simulink model "Bixler"  (R2019b)
settings: Solver=ode45  StartTime=0.0  StopTime=60  RelTol=1e-6  AbsTol=1e-8
PostLoadFcn:
  | parameters_main
  | write_init_cond
StartFcn:
  | write_init_cond
  | disp('Simulating...');
StopFcn:
  | timetime = datestr(datetime('now','Format','hh:mm'));
  | disp(['End of Simulation.       ', timetime]);
  | clear timetime
undefined symbols (not defined in the file): Aero, APlane, Bxl, C, Ctr, deg, DiscIntNeverNeededParam, Earth, F, Guid, Init, Light, MIL, Path, rad, s, Trim, Utility, WGS84
libraries: aerolibconvert2 x39, simulink x14, dspsigops x6, simulink_extras x3, aerolibtransform2 x2, aerolibasang x2, aerolibfltsims x2, shared6dof x1, aerolibadyn x1, aerolibwind2 x1, aerolibanim x1, realtime_pacer_lib x1
(part 1 of 5)
settings Model: SimulationMode=accelerator  PauseTimes=22.8  NumberOfSteps=10  Creator=extra  LastModifiedBy=YK
settings SolverCC: AutoScaleAbsTol=off
settings DataIOCC: SaveFormat=Array  SaveOutput=off  SignalLogging=off  DSMLogging=off  SaveTime=off  ReturnWorkspaceOutputs=off
settings OptimizationCC: EfficientMapNaN2IntZero=off
settings DebuggingCC: ReadBeforeWriteMsg=DisableAll  WriteAfterWriteMsg=DisableAll  WriteAfterReadMsg=DisableAll  MultiTaskDSMMsg=none  ArithmeticOperatorsInVariantConditions=warning
settings HardwareCC: TargetBitPerPointer=64  TargetBitPerSizeT=64  TargetBitPerPtrDiffT=64  TargetLongLongMode=on  TargetIntDivRoundTo=Zero  TargetEndianess=LittleEndian  TargetWordSize=64  TargetHWDeviceType=MATLAB Host  ProdEqTarget=off
settings ModelReferenceCC: UpdateModelReferenceTargets=IfOutOfDate
settings SFSimCC: SimUseLocalCustomCode=off  CustomCodeUndefinedFunction=UseInterfaceOnly
settings RTWCC: RTWUseLocalCustomCode=off
settings CodeAppCC: MaxIdLength=128  StateflowObjectComments=on
settings GRTTargetCC: TargetLangStandard=C89/C90 (ANSI)  CombineOutputUpdateFcns=off  GRTInterface=on
settings SimscapeCC: SimscapeNormalizeSystem=off

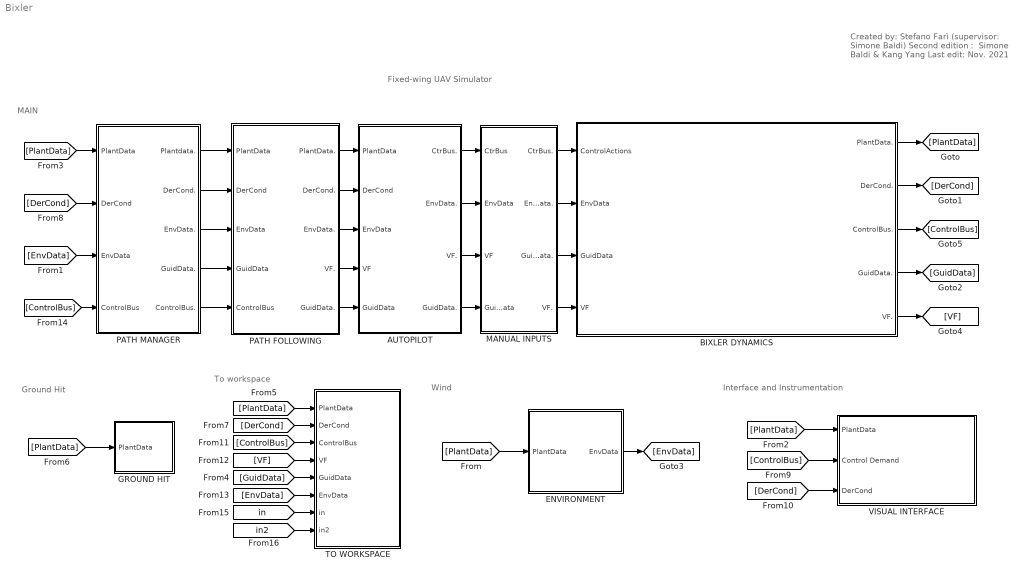
== system Bixler ==
  note: Fixed-wing UAV Simulator
  note: Ground Hit
  note: Interface and Instrumentation
  note: Wind
  note: MAIN
  note: To workspace
  note: Created by: Stefano Farì (supervisor: Simone Baldi)
      | Second edition： Simone Baldi & Kang Yang
      | Last edit: Nov. 2021
  AUTOPILOT : Subsystem
  BIXLER DYNAMICS : Subsystem
      mask Display: image('images/bixler.jpg')
  ENVIRONMENT : Subsystem
  GROUND HIT : Subsystem
  MANUAL INPUTS : Subsystem
  PATH FOLLOWING : Subsystem
  PATH MANAGER : Subsystem
  TO WORKSPACE : Subsystem
  VISUAL INTERFACE : Subsystem
      mask Display: image('images/control_tower.jpg')
  wires:
  BIXLER DYNAMICS/1(PlantData.) -> [PlantData]
  BIXLER DYNAMICS/2(DerCond.) -> [DerCond]
  [PlantData] -> ENVIRONMENT/1(PlantData)
  ENVIRONMENT/1(EnvData) -> [EnvData]
  [PlantData] -> VISUAL INTERFACE/1(PlantData)
  [ControlBus] -> VISUAL INTERFACE/2(Control Demand)
  PATH FOLLOWING/2("DerCond. ") -> AUTOPILOT/2(DerCond)
  PATH FOLLOWING/1("PlantData. ") -> AUTOPILOT/1(PlantData)
  [DerCond] -> VISUAL INTERFACE/3(DerCond)
  MANUAL INPUTS/1(CtrBus.) -> BIXLER DYNAMICS/1(ControlActions)
  [PlantData] -> TO WORKSPACE/1(PlantData)
  [PlantData] -> PATH MANAGER/1(PlantData)
  [DerCond] -> PATH MANAGER/2(DerCond)
  [PlantData] -> GROUND HIT/1(PlantData)
  MANUAL INPUTS/2(EnvData.) -> BIXLER DYNAMICS/2(EnvData)
  [ControlBus] -> TO WORKSPACE/3(ControlBus)
  [DerCond] -> TO WORKSPACE/2(DerCond)
  BIXLER DYNAMICS/3(ControlBus.) -> [ControlBus]
  [EnvData] -> PATH MANAGER/3(EnvData)
  PATH FOLLOWING/4(VF.) -> AUTOPILOT/4(VF)
  PATH FOLLOWING/3(EnvData.) -> AUTOPILOT/3(EnvData)
  PATH FOLLOWING/5(GuidData.) -> AUTOPILOT/5(GuidData)
  AUTOPILOT/4(GuidData.) -> MANUAL INPUTS/4(GuidData)
  BIXLER DYNAMICS/4(GuidData.) -> [GuidData]
  MANUAL INPUTS/3(GuidData.) -> BIXLER DYNAMICS/3(GuidData)
  [GuidData] -> TO WORKSPACE/5(GuidData)
  MANUAL INPUTS/4(VF.) -> BIXLER DYNAMICS/4(VF)
  BIXLER DYNAMICS/5(VF.) -> [VF]
  [VF] -> TO WORKSPACE/4(VF)
  PATH MANAGER/3(EnvData.) -> PATH FOLLOWING/3(EnvData)
  PATH MANAGER/2(DerCond.) -> PATH FOLLOWING/2(DerCond)
  PATH MANAGER/1(Plantdata.) -> PATH FOLLOWING/1(PlantData)
  PATH MANAGER/4(GuidData.) -> PATH FOLLOWING/4(GuidData)
  [EnvData] -> TO WORKSPACE/6(EnvData)
  AUTOPILOT/3(VF.) -> MANUAL INPUTS/3(VF)
  AUTOPILOT/2(EnvData.) -> MANUAL INPUTS/2(EnvData)
  AUTOPILOT/1(CtrBus.) -> MANUAL INPUTS/1(CtrBus)
  [ControlBus] -> PATH MANAGER/4(ControlBus)
  PATH MANAGER/5(ControlBus.) -> PATH FOLLOWING/5(ControlBus)
  [in] -> TO WORKSPACE/7(in)
  [in2] -> TO WORKSPACE/8(in2)

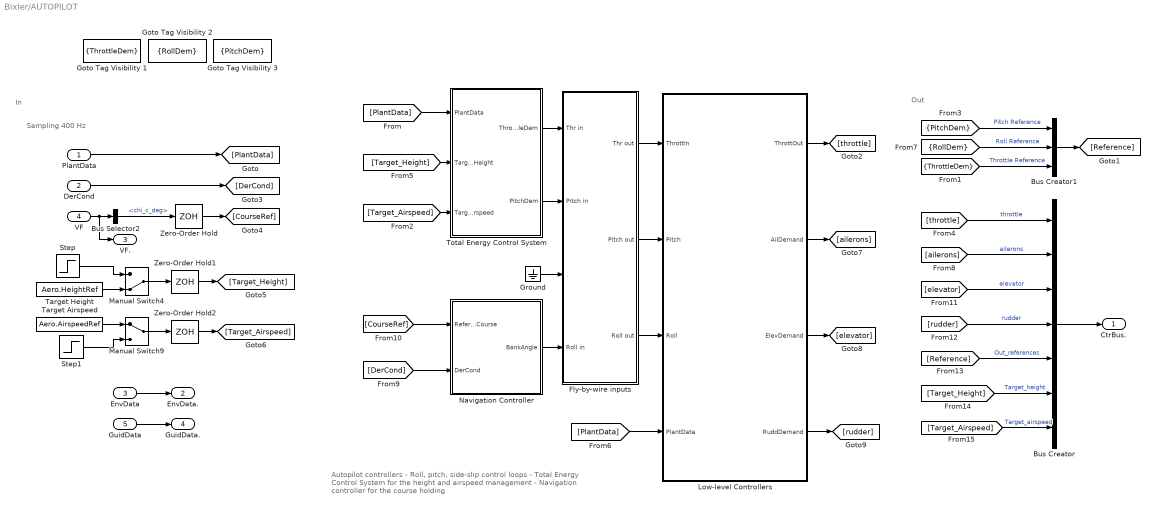
== system Bixler/AUTOPILOT ==
  note: In
  note: Out
  note: Autopilot controllers
      |
      | - Roll, pitch, side-slip control loops
      | - Total Energy Control System for the height and airspeed management
      | - Navigation controller for the course holding
  note: Sampling 400 Hz
  PlantData : Inport
  DerCond : Inport  Port=2
  EnvData : Inport  Port=3
  VF : Inport  Port=4
  GuidData : Inport  Port=5
  Bus Creator : BusCreator  Inputs=7
  Bus Creator1 : BusCreator  Inputs=3
  Bus Selector2 : BusSelector  OutputSignals=chi_c_deg
  Fly-by-wire inputs : Subsystem
  Goto Tag Visibility 1 : GotoTagVisibility  GotoTag=ThrottleDem
  Goto Tag Visibility 2 : GotoTagVisibility  GotoTag=RollDem
  Goto Tag Visibility 3 : GotoTagVisibility  GotoTag=PitchDem
  Ground : Ground
  Low-level Controllers : Subsystem
  Manual Switch4 : ManualSwitch  CurrentSetting=0
  Manual Switch9 : ManualSwitch
  Navigation Controller : Subsystem
  Step : Step  Time=10  Before=50  After=80  SampleTime=0
  Step1 : Step  Time=10  Before=15  After=20  SampleTime=0
  Target Airspeed : Constant  Value=Aero.AirspeedRef
  Target Height : Constant  Value=Aero.HeightRef
  Total Energy Control System : Subsystem
  Zero-Order Hold : ZeroOrderHold  SampleTime=1/400
  Zero-Order Hold1 : ZeroOrderHold  SampleTime=1/400
  Zero-Order Hold2 : ZeroOrderHold  SampleTime=1/400
  CtrBus. : Outport  VectorParamsAs1DForOutWhenUnconnected=off
  EnvData. : Outport  Port=2  VectorParamsAs1DForOutWhenUnconnected=off
  VF. : Outport  Port=3  VectorParamsAs1DForOutWhenUnconnected=off
  GuidData. : Outport  Port=4  VectorParamsAs1DForOutWhenUnconnected=off
  wires:
  Bus Creator1/1 -> [Reference]
  Low-level Controllers/4(RuddDemand) -> [rudder]
  Low-level Controllers/3(ElevDemand) -> [elevator]
  Low-level Controllers/2(AilDemand) -> [ailerons]
  Low-level Controllers/1(ThrottOut) -> [throttle]
  [RollDem] -> Bus Creator1/2  "Roll Reference"
  [CourseRef] -> Navigation Controller/1(ReferenceCourse)
  [PlantData] -> Low-level Controllers/4(PlantData)
  DerCond/1 -> [DerCond]
  [DerCond] -> Navigation Controller/2(DerCond)
  PlantData/1 -> [PlantData]
  Manual Switch4/1 -> Zero-Order Hold1/1
  Manual Switch9/1 -> Zero-Order Hold2/1
  Step/1 -> Manual Switch4/1
  Target Height/1 -> Manual Switch4/2
  Target Airspeed/1 -> Manual Switch9/1
  Step1/1 -> Manual Switch9/2
  [PitchDem] -> Bus Creator1/1  "Pitch Reference"
  Zero-Order Hold/1 -> [CourseRef]
  [PlantData] -> Total Energy Control System/1(PlantData)
  EnvData/1 -> EnvData./1
  GuidData/1 -> GuidData./1
  VF/1 -> VF./1, Bus Selector2/1
  Bus Selector2/1 -> Zero-Order Hold/1  "<chi_c_deg>"
  [ThrottleDem] -> Bus Creator1/3  "Throttle Reference"
  Zero-Order Hold1/1 -> [Target_Height]
  Zero-Order Hold2/1 -> [Target_Airspeed]
  Total Energy Control System/1(ThrottleDem) -> Fly-by-wire inputs/1(Thr in)
  Total Energy Control System/2(PitchDem) -> Fly-by-wire inputs/2(Pitch in)
  Navigation Controller/1(BankAngle) -> Fly-by-wire inputs/4(Roll in)
  Fly-by-wire inputs/1(Thr out) -> Low-level Controllers/1(ThrottIn)
  Fly-by-wire inputs/2(Pitch out) -> Low-level Controllers/2(Pitch)
  Fly-by-wire inputs/3(Roll out) -> Low-level Controllers/3(Roll)
  Ground/1 -> Fly-by-wire inputs/3(.)
  [Target_Height] -> Total Energy Control System/2(Target_Height)
  [Target_Airspeed] -> Total Energy Control System/3(Target_Airspeed)
  [ailerons] -> Bus Creator/2  "ailerons"
  [throttle] -> Bus Creator/1  "throttle"
  [elevator] -> Bus Creator/3  "elevator"
  [rudder] -> Bus Creator/4  "rudder"
  [Reference] -> Bus Creator/5  "Out_references"
  [Target_Height] -> Bus Creator/6  "Target_height"
  [Target_Airspeed] -> Bus Creator/7  "Target_airspeed"
  Bus Creator/1 -> CtrBus./1

== system Bixler/BIXLER DYNAMICS ==
  note: This sub-block contains the dynamics of the aircraft.
      |
      | - All the states and quantities of interest are contained in the Bus signal PlantData.
      | - The derived conditions such as Airspeed, Angle of Attack, and Side-slip angle, are contained in Bus signal DerCond .
      | - The Bus EnvData contains the wind quantities of interest.
      | - The dynamical model is continuous, but the Buses are sampled to feed the discrete-time control system.
      | - The parameters of this block are contained in parameters/parameters_aero.
  ControlActions : Inport
  EnvData : Inport  Port=2
  GuidData : Inport  Port=3
  VF : Inport  Port=4
  Actuator Dynamics : Subsystem
  Bus Selector : BusSelector  OutputSignals=throttle
  RUBBISH BIN : Subsystem
  Sampling : Subsystem
  "Sampling " : Subsystem
  Throttle Dynamics : Subsystem
  Vehicle Airframe : Subsystem
  PlantData. : Outport  VectorParamsAs1DForOutWhenUnconnected=off
  DerCond. : Outport  Port=2  VectorParamsAs1DForOutWhenUnconnected=off
  ControlBus. : Outport  Port=3  VectorParamsAs1DForOutWhenUnconnected=off
  GuidData. : Outport  Port=4  VectorParamsAs1DForOutWhenUnconnected=off
  VF. : Outport  Port=5  VectorParamsAs1DForOutWhenUnconnected=off
  wires:
  Vehicle Airframe/2(DerCond) -> "Sampling "/1(Cont.)  "DerCond"
  Bus Selector/1 -> Throttle Dynamics/1(In)  "<throttle>"
  EnvData/1 -> Vehicle Airframe/3(EnvData)
  ControlActions/1 -> Bus Selector/1, ControlBus./1, Actuator Dynamics/1(In)
  Vehicle Airframe/1(PlantData) -> Sampling/1(Cont.)  "PlantData"
  Sampling/1(Cont.+Disc.) -> PlantData./1
  "Sampling "/1(Cont.+Disc.) -> DerCond./1
  GuidData/1 -> GuidData./1
  VF/1 -> VF./1
  Actuator Dynamics/1(Out) -> Vehicle Airframe/2(ControlActions)
  Throttle Dynamics/1(Out) -> Vehicle Airframe/1(Throttle_cmd)  "throttle"

== system Bixler/ENVIRONMENT ==
  note: Wind slowly time varying
  note: Dynamic wind
  note: Constant wind
  PlantData : Inport
  Bus Creator : BusCreator  Inputs=4
  Bus Selector1 : BusSelector  OutputSignals=xyh,Velocity (inertial),From inertial to body matrix
  Bus Selector2 : BusSelector  OutputSignals=From inertial to body matrix
  Bus Selector3 : BusSelector  OutputSignals=PlantData
  Bus Selector4 : BusSelector  OutputSignals=From inertial to body matrix
  Constant1 : Constant  Value=Init.windConst
  Dot Product : DotProduct  InputSameDT=on  OutDataTypeStr=Inherit: Inherit via internal rule
  Dryden Wind Turbulence Model (Continuous (+q +r)) : aerolibwind2/Dryden Wind Turbulence Model  (Continuous (+q -r))  units=Metric (MKS)  spec=MIL-F-8785C  model=Continuous Dryden (+q +r)  W20=10  Wdeg=135  TurbProb=10^-2 - Light  L_high=533.4  Wingspan=Bxl.b  ts=0.1  Seed=[23341 23342 23343 23344]  T_on=on
  Height : Selector  InputPortWidth=3  IndexOptions=Index vector (dialog)  Indices=3  OutputSizes=1
  Init.DryOnOff : Gain  Gain=Init.DryOnOff
  "Init.DryOnOff " : Gain  Gain=Init.DryOnOff
  Init.WTimevar : Gain  Gain=Init.WTimevar
  Product : Product  Multiplication=Matrix(*)
  "Product " : Product  Multiplication=Matrix(*)
  Slowly time varying wind gen. : Subsystem
  Sum1 : Sum  Inputs=|++
  Sum3 : Sum  Inputs=|++
  Vt : Sqrt  SaturateOnIntegerOverflow=on
  EnvData : Outport  VectorParamsAs1DForOutWhenUnconnected=off
  wires:
  Bus Selector1/1 -> Height/1  "<xyh>"
  Bus Selector1/2 -> Dot Product/2, Dot Product/1  "<Velocity (inertial)>"
  Bus Selector1/3 -> Dryden Wind Turbulence Model (Continuous (+q +r))/3  "<From inertial to body matrix>"
  Bus Selector3/1 -> Bus Selector4/1, Bus Selector1/1, Bus Selector2/1  "<PlantData>"
  Height/1 -> Dryden Wind Turbulence Model (Continuous (+q +r))/1  "Altitude"
  Dot Product/1 -> Vt/1
  Vt/1 -> Dryden Wind Turbulence Model (Continuous (+q +r))/2  "Speed"
  Sum1/1 -> Bus Creator/3, Sum3/2  "Wind velocity (dyn) (body)"
  Constant1/1 -> Product/2
  Bus Creator/1 -> EnvData/1
  "Init.DryOnOff "/1 -> Bus Creator/4  "Wind ang rate (dyn) (body)"
  Sum3/1 -> Bus Creator/2  "Wind total (body)"
  Dryden Wind Turbulence Model (Continuous (+q +r))/1 -> Init.DryOnOff/1
  Bus Selector2/1 -> Product/1  "<From inertial to body matrix>"
  Dryden Wind Turbulence Model (Continuous (+q +r))/2 -> "Init.DryOnOff "/1
  PlantData/1 -> Bus Selector3/1
  Product/1 -> Bus Creator/1, Sum3/1  "Wind velocity (sta) (body)"
  Bus Selector4/1 -> "Product "/1  "<From inertial to body matrix>"
  Init.WTimevar/1 -> Sum1/2  "Wind slowly time varying"
  Init.DryOnOff/1 -> Sum1/1
  "Product "/1 -> Init.WTimevar/1
  Slowly time varying wind gen./1(Out1) -> "Product "/2

== system Bixler/GROUND HIT ==
  PlantData : Inport
  Bus Selector1 : BusSelector  OutputSignals=PlantData.xyh
  Constant : Constant  Value=0
  Relational Operator : RelationalOperator  Operator=<=  OutDataTypeStr=boolean  RndMeth=Simplest
  Selector : Selector  InputPortWidth=3  IndexOptions=Index vector (dialog)  Indices=3  OutputSizes=1
  Stop Simulation : Stop
  wires:
  Selector/1 -> Relational Operator/1
  Bus Selector1/1 -> Selector/1  "<xyh>"
  Constant/1 -> Relational Operator/2
  Relational Operator/1 -> Stop Simulation/1
  PlantData/1 -> Bus Selector1/1

== system Bixler/MANUAL INPUTS ==
  note: Manual control
      |
      | The switches below enable (up position) or disable (down position) the manual control in the Visual Interface sub-block.
      | (default: down)
  note: Open-loop inputs
      |
      | The switches below enables a custom input from the Workspace (timeseries data type) to the control surfaces.
  note: Trim condition
      |
      | The sub-block below allows to try the actuators configuration for a trimmed flight.
  CtrBus : Inport
  EnvData : Inport  Port=2
  VF : Inport  Port=3
  GuidData : Inport  Port=4
  Bus Creator : BusCreator  Inputs=7
  Bus Selector : BusSelector  OutputSignals=throttle,ailerons,elevator,rudder
  Bus Selector1 : BusSelector  OutputSignals=Out_references,Target_height,Target_airspeed
  "CtrBus " : InportShadow
  From Workspace1 : FromWorkspace  Commented=on  VariableName=LogData.RCIN.ElevDem_IN  SampleTime=0.001
  From Workspace2 : FromWorkspace  Commented=on  VariableName=LogData.RCIN.RuddDem_IN  SampleTime=0.001
  From Workspace3 : FromWorkspace  Commented=on  VariableName=LogData.RCIN.ThrottleDem_IN  SampleTime=0.001
  From Workspace4 : FromWorkspace  Commented=on  VariableName=LogData.RCIN.AilDem_IN  SampleTime=0.001
  Goto4 : Goto  Commented=on  GotoTag=throttle
  Manual Switch{,1..7} (8 alike) : ManualSwitch  CurrentSetting=0
  Manual_cmd{,4..6} (4 alike) : Constant  Value=0
  Trim conditions : Subsystem
  CtrBus. : Outport  VectorParamsAs1DForOutWhenUnconnected=off
  EnvData. : Outport  Port=2  VectorParamsAs1DForOutWhenUnconnected=off
  GuidData. : Outport  Port=3  VectorParamsAs1DForOutWhenUnconnected=off
  VF. : Outport  Port=4  VectorParamsAs1DForOutWhenUnconnected=off
  wires:
  Manual Switch4/1 -> Goto4/1, Bus Creator/1  "throttle"
  Manual Switch7/1 -> Bus Creator/3  "elevator"
  Manual_cmd/1 -> Manual Switch/1
  Manual_cmd4/1 -> Manual Switch1/1
  Manual Switch5/1 -> Bus Creator/2  "ailerons"
  Manual Switch6/1 -> Bus Creator/4  "rudder"
  Manual_cmd6/1 -> Manual Switch3/1
  Manual_cmd5/1 -> Manual Switch2/1
  Bus Creator/1 -> CtrBus./1
  Manual Switch1/1 -> Manual Switch5/2  "ailerons"
  Manual Switch2/1 -> Manual Switch7/2  "elevator"
  Manual Switch3/1 -> Manual Switch6/2  "rudder"
  From Workspace3/1 -> Manual Switch4/1
  Manual Switch/1 -> Manual Switch4/2
  Bus Selector/1 -> Trim conditions/1(throttle)  "<throttle>"
  Trim conditions/1(throttout) -> Manual Switch/2
  Bus Selector/2 -> Trim conditions/2(ail)  "<ailerons>"
  Bus Selector/3 -> Trim conditions/3(elev)  "<elevator>"
  Bus Selector/4 -> Trim conditions/4(rudd)  "<rudder>"
  Trim conditions/4(ruddout) -> Manual Switch3/2
  Trim conditions/2(ailout) -> Manual Switch1/2
  Trim conditions/3(elevout) -> Manual Switch2/2
  EnvData/1 -> EnvData./1
  From Workspace4/1 -> Manual Switch5/1
  From Workspace1/1 -> Manual Switch7/1
  From Workspace2/1 -> Manual Switch6/1
  GuidData/1 -> GuidData./1
  VF/1 -> VF./1
  CtrBus/1 -> Bus Selector/1
  "CtrBus "/1 -> Bus Selector1/1
  Bus Selector1/1 -> Bus Creator/5  "<Out_references>"
  Bus Selector1/2 -> Bus Creator/6  "<Target_height>"
  Bus Selector1/3 -> Bus Creator/7  "<Target_airspeed>"

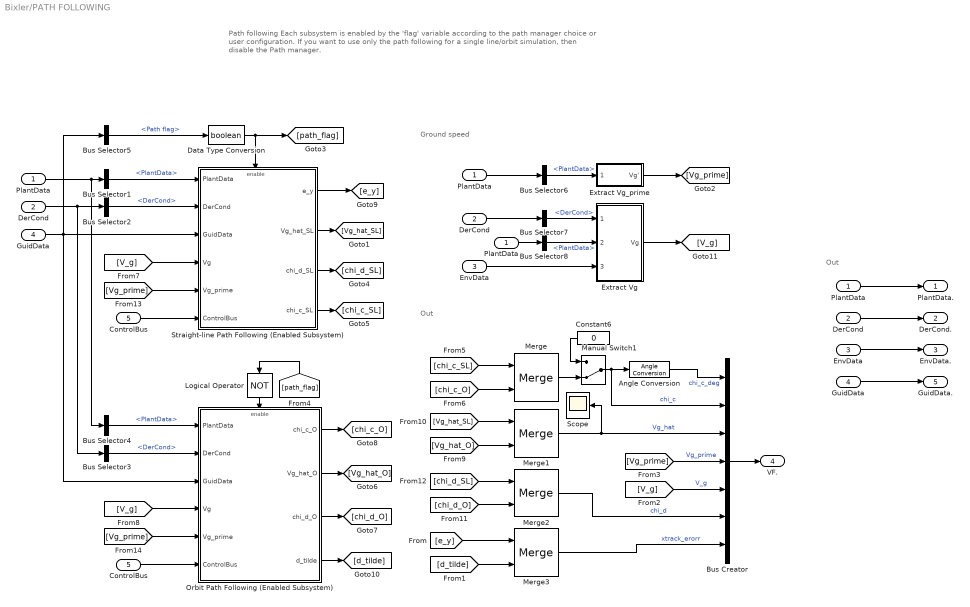
== system Bixler/PATH FOLLOWING ==
  note: Out
  note: Ground speed
  note: Out
  note: Path following
      |
      | Each subsystem is enabled by the 'flag' variable according to the path manager choice or user configuration.
      | If you want to use only the path following for a single line/orbit simulation, then disable the Path manager.
  PlantData : Inport
  DerCond : Inport  Port=2
  EnvData : Inport  Port=3
  GuidData : Inport  Port=4
  ControlBus : Inport  Port=5
  Angle Conversion : aerolibconvert2/Angle Conversion  IU=rad  OU=deg
  Bus Creator : BusCreator  Inputs=7
  Bus Selector{1,4,6,8} (4 alike) : BusSelector  OutputSignals=PlantData
  Bus Selector2 : BusSelector  OutputSignals=DerCond
  Bus Selector3 : BusSelector  OutputSignals=DerCond
  Bus Selector5 : BusSelector  OutputSignals=Path flag
  Bus Selector7 : BusSelector  OutputSignals=DerCond
  Constant6 : Constant  Value=0
  "ControlBus " : InportShadow  Port=5
  Data Type Conversion : DataTypeConversion  OutDataTypeStr=boolean
  "DerCond " : InportShadow  Port=2
  "DerCond  " : InportShadow  Port=2
  "EnvData " : InportShadow  Port=3
  Extract Vg : Subsystem
  Extract Vg_prime : Subsystem
  "GuidData " : InportShadow  Port=4
  Logical Operator : Logic  Operator=NOT  AllPortsSameDT=off  OutDataTypeStr=boolean
  Manual Switch1 : ManualSwitch  CurrentSetting=0
  Merge{,1..3} (4 alike) : Merge
  Orbit Path Following (Enabled Subsystem) : Subsystem  TreatAsAtomicUnit=on
  "PlantData " : InportShadow
  "PlantData  " : InportShadow
  "PlantData   " : InportShadow
  Scope : Scope
  Straight-line Path Following (Enabled Subsystem) : Subsystem  TreatAsAtomicUnit=on
  "PlantData. " : Outport  VectorParamsAs1DForOutWhenUnconnected=off
  "DerCond. " : Outport  Port=2  VectorParamsAs1DForOutWhenUnconnected=off
  EnvData. : Outport  Port=3  VectorParamsAs1DForOutWhenUnconnected=off
  VF. : Outport  Port=4  VectorParamsAs1DForOutWhenUnconnected=off
  GuidData. : Outport  Port=5  VectorParamsAs1DForOutWhenUnconnected=off
  wires:
  Merge/1 -> Manual Switch1/2
  Constant6/1 -> Manual Switch1/1
  EnvData/1 -> EnvData./1
  PlantData/1 -> Bus Selector4/1, Bus Selector1/1
  Bus Selector1/1 -> Straight-line Path Following (Enabled Subsystem)/1(PlantData)  "<PlantData>"
  DerCond/1 -> Bus Selector2/1, Bus Selector3/1
  Bus Creator/1 -> VF./1
  Manual Switch1/1 -> Bus Creator/2, Angle Conversion/1  "chi_c"
  Logical Operator/1 -> Orbit Path Following (Enabled Subsystem)/Enable
  Bus Selector4/1 -> Orbit Path Following (Enabled Subsystem)/1(PlantData)  "<PlantData>"
  Bus Selector3/1 -> Orbit Path Following (Enabled Subsystem)/2(DerCond)  "<DerCond>"
  Data Type Conversion/1 -> [path_flag], Straight-line Path Following (Enabled Subsystem)/Enable
  [path_flag] -> Logical Operator/1
  Bus Selector2/1 -> Straight-line Path Following (Enabled Subsystem)/2(DerCond)  "<DerCond>"
  Merge1/1 -> Bus Creator/3, Scope/1  "Vg_hat"
  [Vg_prime] -> Bus Creator/4  "Vg_prime"
  Straight-line Path Following (Enabled Subsystem)/2(Vg_hat_SL) -> [Vg_hat_SL]
  Straight-line Path Following (Enabled Subsystem)/3(chi_d_SL) -> [chi_d_SL]
  Straight-line Path Following (Enabled Subsystem)/4(chi_c_SL) -> [chi_c_SL]
  Orbit Path Following (Enabled Subsystem)/2(Vg_hat_O) -> [Vg_hat_O]
  Orbit Path Following (Enabled Subsystem)/3(chi_d_O) -> [chi_d_O]
  Orbit Path Following (Enabled Subsystem)/1(chi_c_O) -> [chi_c_O]
  [chi_c_SL] -> Merge/1
  [chi_c_O] -> Merge/2
  [Vg_hat_O] -> Merge1/2
  [Vg_hat_SL] -> Merge1/1
  [chi_d_O] -> Merge2/2
  [chi_d_SL] -> Merge2/1
  Merge2/1 -> Bus Creator/6  "chi_d"
  Angle Conversion/1 -> Bus Creator/1  "chi_c_deg"
  Straight-line Path Following (Enabled Subsystem)/1(e_y) -> [e_y]
  [e_y] -> Merge3/1
  Orbit Path Following (Enabled Subsystem)/4(d_tilde) -> [d_tilde]
  [d_tilde] -> Merge3/2
  Merge3/1 -> Bus Creator/7  "xtrack_erorr"
  GuidData/1 -> Orbit Path Following (Enabled Subsystem)/3(GuidData), Straight-line Path Following (Enabled Subsystem)/3(GuidData), Bus Selector5/1
  Bus Selector5/1 -> Data Type Conversion/1  "<Path flag>"
  "DerCond "/1 -> "DerCond. "/1
  "GuidData "/1 -> GuidData./1
  "PlantData "/1 -> "PlantData. "/1
  Extract Vg_prime/1(Vg') -> [Vg_prime]
  Bus Selector6/1 -> Extract Vg_prime/1(PlantData)  "<PlantData>"
  [V_g] -> Bus Creator/5  "V_g"
  Extract Vg/1(Vg) -> [V_g]
  "PlantData  "/1 -> Bus Selector6/1
  "DerCond  "/1 -> Bus Selector7/1
  Bus Selector7/1 -> Extract Vg/1(DerCond)  "<DerCond>"
  [V_g] -> Straight-line Path Following (Enabled Subsystem)/4(Vg)
  [V_g] -> Orbit Path Following (Enabled Subsystem)/4(Vg)
  [Vg_prime] -> Straight-line Path Following (Enabled Subsystem)/5(Vg_prime)
  [Vg_prime] -> Orbit Path Following (Enabled Subsystem)/5(Vg_prime)
  "EnvData "/1 -> Extract Vg/3(Envdata)
  ControlBus/1 -> Straight-line Path Following (Enabled Subsystem)/6(ControlBus)
  "ControlBus "/1 -> Orbit Path Following (Enabled Subsystem)/6(ControlBus)
  "PlantData   "/1 -> Bus Selector8/1
  Bus Selector8/1 -> Extract Vg/2(PlantData)  "<PlantData>"

== system Bixler/PATH MANAGER ==
  note: Change this switch to enable/disable the path manager (down = disabled).
  note: Path following only
  note: Path manager
  PlantData : Inport
  DerCond : Inport  Port=2
  EnvData : Inport  Port=3
  ControlBus : Inport  Port=4
  Bus Creator1 : BusCreator  Inputs=6
  Bus Creator2 : BusCreator  Inputs=6
  Bus Selector : BusSelector  OutputSignals=PlantData.Position (inertial)
  Constant1 : Constant  Value=Guid.SL.Line_Origin
  Constant10 : Constant  Value=Path.waypoints
  Constant2 : Constant  Value=Guid.Loiter.R
  Constant3 : Constant  Value=Guid.Loiter.R
  Constant4 : Constant  Value=Guid.SL.Line_Slope
  Constant5 : Constant  Value=Guid.Loiter.R
  Constant6 : Constant  Value=Guid.Loiter.C
  Constant7 : Constant  Value=Guid.Loiter.j
  Constant8 : Constant  Value=Guid.Strategy
  Demux : Demux  Outputs=2
  Manual Switch : ManualSwitch  CurrentSetting=0
  Path Manager : MATLAB Function  Commented=on  TreatAsAtomicUnit=on
  Scope : Scope
  Scope1 : Scope
  Selector2 : Selector  InputPortWidth=3  IndexOptions=Index vector (dialog)  Indices=[1 2]  OutputSizes=1
  Stop Simulation : Stop
  Plantdata. : Outport  VectorParamsAs1DForOutWhenUnconnected=off
  DerCond. : Outport  Port=2  VectorParamsAs1DForOutWhenUnconnected=off
  EnvData. : Outport  Port=3  VectorParamsAs1DForOutWhenUnconnected=off
  GuidData. : Outport  Port=4  VectorParamsAs1DForOutWhenUnconnected=off
  ControlBus. : Outport  Port=5  VectorParamsAs1DForOutWhenUnconnected=off
  wires:
  Constant8/1 -> Bus Creator1/1  "Path flag"
  Constant1/1 -> Bus Creator1/2  "SL_Origin"
  Constant4/1 -> Bus Creator1/3  "SL_Slope"
  Constant6/1 -> Bus Creator1/4  "Orbit_C"
  Constant5/1 -> Bus Creator1/5  "Orbit_R"
  Constant7/1 -> Bus Creator1/6  "Orbit_j"
  PlantData/1 -> Bus Selector/1, Plantdata./1
  DerCond/1 -> DerCond./1
  EnvData/1 -> EnvData./1
  Constant10/1 -> Path Manager/1(w)
  Bus Selector/1 -> Selector2/1  "<Position (inertial)>"
  Demux/1 -> Path Manager/2(x)
  Path Manager/6(stop_sim) -> Stop Simulation/1
  Selector2/1 -> Demux/1
  Demux/2 -> Path Manager/3(y)
  Bus Creator1/1 -> Manual Switch/2
  Manual Switch/1 -> GuidData./1
  Path Manager/7(z) -> Scope1/1
  Constant2/1 -> Path Manager/4(R)
  Bus Creator2/1 -> Manual Switch/1
  Path Manager/1(flag) -> Scope/1, Bus Creator2/1  "Path flag"
  Path Manager/2(origin) -> Bus Creator2/2  "SL_Origin"
  Path Manager/3(slope) -> Bus Creator2/3  "SL_Slope"
  Path Manager/4(c) -> Bus Creator2/4  "Orbit_C"
  Constant3/1 -> Bus Creator2/5  "Orbit_R"
  Path Manager/5(lambda) -> Bus Creator2/6  "Orbit_j"
  ControlBus/1 -> ControlBus./1

== system Bixler/TO WORKSPACE ==
  PlantData : Inport
  DerCond : Inport  Port=2
  ControlBus : Inport  Port=3
  VF : Inport  Port=4
  GuidData : Inport  Port=5
  EnvData : Inport  Port=6
  in : Inport  Port=7
  in2 : Inport  Port=8
  Bus Creator : BusCreator  Inputs=8
  Bus Selector4 : BusSelector  OutputSignals=DerCond
  Bus Selector5 : BusSelector  OutputSignals=PlantData
  Sample at 0.01s : ZeroOrderHold  SampleTime=0.01
  To Workspace2 : ToWorkspace  VariableName=SimOut  SaveFormat=Timeseries  SampleTime=-1
      settings: Save2DSignal=2-D array (concatenate along first dimension)
  wires:
  Bus Creator/1 -> Sample at 0.01s/1
  Bus Selector5/1 -> Bus Creator/1  "<PlantData>"
  PlantData/1 -> Bus Selector5/1
  ControlBus/1 -> Bus Creator/3  "ControlBus"
  DerCond/1 -> Bus Selector4/1
  Bus Selector4/1 -> Bus Creator/2  "<DerCond>"
  GuidData/1 -> Bus Creator/5  "GuidData"
  VF/1 -> Bus Creator/4  "VF"
  EnvData/1 -> Bus Creator/6  "EnvData"
  Sample at 0.01s/1 -> To Workspace2/1
  in/1 -> Bus Creator/7
  in2/1 -> Bus Creator/8

== system Bixler/VISUAL INTERFACE ==
  note: Position[m]:&nbsp;&nbsp;&nbsp;&nbsp;&nbsp;&nbsp;&nbsp;&nbsp;&nbsp;&nbsp;&nbsp;&nbsp;&nbsp;&nbsp;&nbsp;[0 0 -50]<br>Velocity[m/s]:&nbsp;&nbsp;&nbsp;&nbsp;&nbsp;&nbsp;&nbsp;&nbsp;&nbsp;&nbsp;&nbsp;&nbsp;&nbsp;[15 0 0]<br>Attitude[deg]:&nbsp;&nbsp;&nbsp;&nbsp;&nbsp;&nbsp;&nbsp;&nbsp;&nbsp;&nbsp;&nbsp;&nbsp;&nbsp;[0 0 0]<br>Angular rates[deg/s]:&nbsp;[0 0 0]<br><br>W. amplitude[m/s]:&nbsp;&nbsp;&nbsp;&nbsp;[-2 -3.4641 0]<br>
  note: Initial conditions
      | (Updates automatically)
  note: Extract data
  note: (remember to change the switch positions in the main block and to slow down the simulation with the Real-Time Parser)
  note: Actuators
  note: Positive, nose left-yawing
  note: Positive, right wing down
  note: Positive, nose down
  note: RUDDER
  note: AILERONS
  note: THROTTLE
  note: [m/s]
  note: [m]
  note: [m/s]
  note: ELEVATOR
  note: Slow down simulation to match
      | with real clock time
  PlantData : Inport
  Control Demand : Inport  Port=2
  DerCond : Inport  Port=3
  Ailerons : Display
  Airspeed Indicator : AirspeedIndicatorBlock  LabelPosition=Hide  ScaleMin=0  ScaleMax=40
  Altimeter : AltimeterBlock  LabelPosition=Hide
  Artificial Horizon : ArtificialHorizonBlock  LabelPosition=Hide
  Bus Selector : BusSelector  OutputSignals=Position (inertial),Euler angles (rad)
  Bus Selector1 : BusSelector  OutputSignals=PlantData
  Bus Selector2 : BusSelector  OutputSignals=DerCond
  Climb Rate Indicator : ClimbIndicatorBlock  LabelPosition=Hide  ScaleMax=20000
  Data for instrumentation below : Subsystem
  Elevator : Display
  Half Gauge : SemiCircularGaugeBlock  ScaleMin=-30  ScaleMax=30
  Half Gauge1 : SemiCircularGaugeBlock  ScaleMin=-30  ScaleMax=30
  Half Gauge2 : SemiCircularGaugeBlock  ScaleMin=-30  ScaleMax=30
  Half Gauge3 : SemiCircularGaugeBlock
  Heading Indicator : HeadingIndicatorBlock  LabelPosition=Hide
  MATLAB Animation : aerolibanim/MATLAB Animation  Tag=Matlab Animation 6 DOF  Vehicles=1  Geometries='astredwedge.mat'  BoundingBoxCoordinates=[-50,50,-50,50,-50,50]  CameraOffset=[-150,-50,0]  CameraViewAngle=3  SampleTime=0.2  FigurePosition=[6.189552e+01,5.544776e+01,6.039403e+02,5.444776e+02]
      settings: SourceProductBaseCode=AE
  Real-Time Pacer : realtime_pacer_lib/Real-Time Pacer  simTimePerRealTime=inf
  Rudder : Display
  Slider : SliderBlock
  Slider1 : SliderBlock  ScaleMin=-2  ScaleMax=2  TickInterval=1
  Slider2 : SliderBlock  ScaleMin=-1  ScaleMax=1  TickInterval=0.2
  Slider3 : SliderBlock  ScaleMin=-1  ScaleMax=1  TickInterval=0.2
  Subsystem : Subsystem
  Throttle : Display
  To FlightGear : Subsystem  Commented=on
  wires:
  Bus Selector/1 -> To FlightGear/1(In1), MATLAB Animation/1  "<Position (inertial)>"
  Bus Selector1/1 -> Data for instrumentation below/1(PlantData), Bus Selector/1  "<PlantData>"
  Bus Selector/2 -> To FlightGear/2(In2), MATLAB Animation/2  "<Euler angles (rad)>"
  Control Demand/1 -> Subsystem/1(Control Demand)
  Subsystem/1(t) -> Throttle/1
  Subsystem/2(e) -> Elevator/1
  Subsystem/3(a) -> Ailerons/1
  Subsystem/4(r) -> Rudder/1
  DerCond/1 -> Bus Selector2/1
  PlantData/1 -> Bus Selector1/1
  Bus Selector2/1 -> Data for instrumentation below/2(DerCond)  "<DerCond>"

== system Bixler/AUTOPILOT/Fly-by-wire inputs ==
  note: Put here your custom inputs
  Thr in : Inport
  Pitch in : Inport  Port=2
  . : Inport  Port=3
  Roll in : Inport  Port=4
  Constant : Constant  Commented=on  Value=0
  Dummy port : Terminator
  From Workspace : FromWorkspace  Commented=on  VariableName=LogData.RCIN.Throttle_IN  SampleTime=0.001
  From Workspace1 : FromWorkspace  Commented=on  VariableName=LogData.RCIN.Pitch_IN  SampleTime=0.001
  From Workspace2 : FromWorkspace  Commented=on  VariableName=LogData.RCIN.Roll_IN  SampleTime=0.001
  Manual Switch1 : ManualSwitch  CurrentSetting=0
  Manual Switch2 : ManualSwitch
  Manual Switch3 : ManualSwitch
  Manual Switch4 : ManualSwitch
  Thr out : Outport  VectorParamsAs1DForOutWhenUnconnected=off
  Pitch out : Outport  Port=2  VectorParamsAs1DForOutWhenUnconnected=off
  Roll out : Outport  Port=3  VectorParamsAs1DForOutWhenUnconnected=off
  tag scope: PitchDem=scoped, RollDem=scoped, ThrottleDem=scoped
  wires:
  Manual Switch3/1 -> Pitch out/1
  Manual Switch1/1 -> Thr out/1
  Pitch in/1 -> [PitchDem], Manual Switch3/1
  From Workspace/1 -> Manual Switch1/1
  Manual Switch2/1 -> [RollDem], Roll out/1
  Roll in/1 -> Manual Switch2/1
  From Workspace1/1 -> Manual Switch3/2
  Thr in/1 -> [ThrottleDem], Manual Switch1/2
  Constant/1 -> Manual Switch4/2
  From Workspace2/1 -> Manual Switch4/1
  Manual Switch4/1 -> Manual Switch2/2
  ./1 -> Dummy port/1

== system Bixler/AUTOPILOT/Low-level Controllers ==
  ThrottIn : Inport  Unit=%
  Pitch : Inport  Port=2  Unit=deg
  Roll : Inport  Port=3  Unit=deg
  PlantData : Inport  Port=4
  Angle Conversion1 : aerolibconvert2/Angle Conversion  IU=rad  OU=deg
  Angle Conversion2 : aerolibconvert2/Angle Conversion  IU=rad  OU=deg
  Angular Velocity Conversion : aerolibconvert2/Angular Velocity Conversion  IU=rad/s  OU=deg/s
  Angular Velocity Conversion1 : aerolibconvert2/Angular Velocity Conversion  IU=rad/s  OU=deg/s
  Bus Selector : BusSelector  OutputSignals=PlantData.Euler angles (rad)
  Bus Selector1 : BusSelector  OutputSignals=PlantData.Angular rates (body) (rad/s)
  Bus Selector2 : BusSelector  OutputSignals=PlantData.Euler angles (rad)
  Bus Selector3 : BusSelector  OutputSignals=PlantData.Angular rates (body) (rad/s)
  Bus Selector5 : BusSelector  OutputSignals=PlantData.Angular rates (body) (rad/s)
  Bus Selector6 : BusSelector  OutputSignals=PlantData.Euler angles (rad)
  Bus Selector7 : BusSelector  OutputSignals=PlantData.Accelerations (body/body)
  Get scaling factor : Subsystem
  Pitch controller : Subsystem
  Roll controller : Subsystem
  Side-slip angle controller : Subsystem
  ThrottOut : Outport  Unit=%  VectorParamsAs1DForOutWhenUnconnected=off
  AilDemand : Outport  Port=2  Unit=deg  VectorParamsAs1DForOutWhenUnconnected=off
  ElevDemand : Outport  Port=3  Unit=deg  VectorParamsAs1DForOutWhenUnconnected=off
  RuddDemand : Outport  Port=4  Unit=deg  VectorParamsAs1DForOutWhenUnconnected=off
  wires:
  Bus Selector/1 -> Angle Conversion1/1  "<Euler angles (rad)>"
  Roll controller/1(AilDemand) -> [AilDem], AilDemand/1
  Bus Selector1/1 -> Angular Velocity Conversion1/1  "<Angular rates (body) (rad/s)>"
  Bus Selector2/1 -> Angle Conversion2/1  "<Euler angles (rad)>"
  Bus Selector3/1 -> Angular Velocity Conversion/1  "<Angular rates (body) (rad/s)>"
  Pitch controller/1(ElevDemand) -> ElevDemand/1
  Get scaling factor/1(Scaler) -> Roll controller/4(Scaler), Side-slip angle controller/4(Scaler), Pitch controller/4(Scaler)
  Bus Selector7/1 -> Side-slip angle controller/3(accel_y)  "<Accelerations (body/body)>"
  Bus Selector6/1 -> Side-slip angle controller/2("Euler angles ")  "<Euler angles (rad)>"
  Bus Selector5/1 -> Side-slip angle controller/1(Yaw_rate)  "<Angular rates (body) (rad/s)>"
  [PlantData] -> Bus Selector1/1, Bus Selector2/1, Bus Selector3/1, Bus Selector5/1, Bus Selector6/1, Bus Selector7/1, Bus Selector/1
  Pitch/1 -> [PitchRef]
  PlantData/1 -> [PlantData]
  ThrottIn/1 -> ThrottOut/1
  Angle Conversion2/1 -> Pitch controller/2(EulerAngles)
  Angular Velocity Conversion/1 -> Pitch controller/3(AngularRates)
  Angle Conversion1/1 -> Roll controller/2(Euler angles)
  Angular Velocity Conversion1/1 -> Roll controller/3(AngularRates)
  Roll/1 -> [RollRef]
  [PitchRef] -> Pitch controller/1(PitchReference)
  [RollRef] -> Roll controller/1(RollReference)
  [AilDem] -> Side-slip angle controller/5(AilDemand)
  Side-slip angle controller/1(RudderDemand) -> RuddDemand/1

== system Bixler/AUTOPILOT/Navigation Controller ==
  ReferenceCourse : Inport  Unit=deg
  DerCond : Inport  Port=2
  Angle Conversion : aerolibconvert2/Angle Conversion  IU=rad  OU=deg
  Bus Selector : BusSelector  OutputSignals=DerCond.Course
  Constant : Constant  Value=45
  Discrete PID Controller : simulink/Continuous/PID Controller  Controller=PD  Form=Parallel  TimeDomain=Discrete-time  SampleTime=Ctr.TS  IntegratorMethod=Forward Euler  FilterMethod=Forward Euler  ControllerParametersSource=internal  P=Ctr.Hdg2Roll.NAV_ROLL_P  I=0.01  D=Ctr.Hdg2Roll.NAV_ROLL_D  UseFilter=on  N=2*pi*20  TunerSelectOption=Transfer Function Based (PID Tuner App)  InitialConditionSource=internal  InitialConditionForIntegrator=0  InitialConditionForFilter=0  DifferentiatorICPrevScaledInput=0  ExternalReset=none  TrackingMode=off  Kt=1  LimitOutput=on  UpperSaturationLimit=45  LowerSaturationLimit=-45  LinearizeAsGain=off  AntiWindupMode=clamping  Kb=1  POutMin=[]  POutMax=[]  IOutMin=[]  IOutMax=[]  DOutMin=[]  DOutMax=[]  NOutMin=[]  NOutMax=[]  SumOutMin=[]  SumOutMax=[]  SaturationOutMin=[]  SaturationOutMax=[]  PParamMin=[]  PParamMax=[]  IParamMin=[]  IParamMax=[]  DParamMin=[]  DParamMax=[]  NParamMin=[]  NParamMax=[]  KbParamMin=[]  KbParamMax=[]  KtParamMin=[]  KtParamMax=[]  KbOutMin=[]  KbOutMax=[]  KtOutMin=[]  KtOutMax=[]  IntegratorOutMin=[]  IntegratorOutMax=[]  FilterOutMin=[]  FilterOutMax=[]  SumI1OutMin=[]  SumI1OutMax=[]  SumI2OutMin=[]  SumI2OutMax=[]  SumI3OutMin=[]  SumI3OutMax=[]  SumI4OutMin=[]  SumI4OutMax=[]  SumDOutMin=[]  SumDOutMax=[]  DifferentiatorOutMin=[]  DifferentiatorOutMax=[]  FilterDiffOutCoefMin=[]  FilterDiffOutCoefMax=[]  ReciprocalOutMin=[]  ReciprocalOutMax=[]  SumDenOutMin=[]  SumDenOutMax=[]  SumNumOutMin=[]  SumNumOutMax=[]  DivideOutMin=[]  DivideOutMax=[]  IntegratorContinuousStateAttributes=''  IntegratorStateMustResolveToSignalObject=off  IntegratorRTWStateStorageClass=Auto  FilterContinuousStateAttributes=''  FilterStateMustResolveToSignalObject=off  FilterRTWStateStorageClass=Auto  ParallelPVariant=InternalParameters  IdealPVariant=Disabled  IVariant=Disabled  DVariant=InternalParameters  IntegratorVariant=Disabled  SatVariant=Enabled  AWVariant=Disabled  PCopyVariant=Disabled  TRVariant=Disabled  FdbkBlocksVariant=Forward  IdealPFdbkVariant=Disabled  SatFdbkVariant=Disabled  DerivativeFilterVariant=ForwardEulerFilter  NVariant=InternalParameters  NCopyVariant=Disabled  FilterICVariant=InternalICsFilter  IntegratorICVariant=Disabled  ExternalResetVariant=Disabled  TRSumVariant=Passthrough  SumFdbkVariant=Disabled  SumVariant=Sum_PD
  Manual Switch : ManualSwitch  CurrentSetting=0
  Manual Switch1 : ManualSwitch
  PID : Subsystem  Commented=on
  Scope : Scope
  Scope1 : Scope
  Scope2 : Scope  NumInputPorts=2
  Step : Step  Time=10  After=90  SampleTime=0
  Sum : Sum  Inputs=|+-
  Unwrap : Subsystem
  Unwrap1 : dspsigops/Unwrap  tol=pi  InputProcessing=Columns as channels (frame based)  running=off
  Zero-Order Hold : ZeroOrderHold  SampleTime=1/400
  BankAngle : Outport  Unit=deg  VectorParamsAs1DForOutWhenUnconnected=off
  wires:
  Bus Selector/1 -> Unwrap1/1  "<Course>"
  Discrete PID Controller/1 -> Manual Switch1/1, Scope/1
  DerCond/1 -> Bus Selector/1
  Unwrap1/1 -> Angle Conversion/1  "chi_measured"
  Sum/1 -> Scope1/1, Discrete PID Controller/1
  Angle Conversion/1 -> Sum/2, Scope2/2
  ReferenceCourse/1 -> Manual Switch/2
  Unwrap/1(Out) -> Scope2/1, Sum/1
  Manual Switch/1 -> Unwrap/1(In)
  Step/1 -> Zero-Order Hold/1
  Zero-Order Hold/1 -> Manual Switch/1
  Manual Switch1/1 -> BankAngle/1
  Constant/1 -> Manual Switch1/2

== system Bixler/AUTOPILOT/Total Energy Control System ==
  note: TECS (Total Energy Control System)
      |
      | It is meant to solve the cross-coupling between height and airspeed control. This is a simplified version of the TECS (see thesis for details). This implementation has the same theoretical behaviour of ArduPilot, but without a direct correspondence with its parameters.
  PlantData : Inport
  Target_Height : Inport  Port=2
  Target_Airspeed : Inport  Port=3
  Bus Selector1 : BusSelector  OutputSignals=PlantData.xyh
  Discrete PID Controller 1 : simulink/Continuous/PID Controller  Controller=PID  Form=Parallel  TimeDomain=Discrete-time  SampleTime=Ctr.TS  IntegratorMethod=Forward Euler  FilterMethod=Forward Euler  ControllerParametersSource=internal  P=1.73635676332661  I=0.34363794334664  D=0.534286386520939  UseFilter=on  N=1.11842208231346  TunerSelectOption=Transfer Function Based (PID Tuner App)  InitialConditionSource=internal  InitialConditionForIntegrator=0  InitialConditionForFilter=0  DifferentiatorICPrevScaledInput=0  ExternalReset=none  TrackingMode=off  Kt=1  LimitOutput=on  UpperSaturationLimit=100  LowerSaturationLimit=0  LinearizeAsGain=off  AntiWindupMode=clamping  Kb=1  POutMin=[]  POutMax=[]  IOutMin=[]  IOutMax=[]  DOutMin=[]  DOutMax=[]  NOutMin=[]  NOutMax=[]  SumOutMin=[]  SumOutMax=[]  SaturationOutMin=[]  SaturationOutMax=[]  PParamMin=[]  PParamMax=[]  IParamMin=[]  IParamMax=[]  DParamMin=[]  DParamMax=[]  NParamMin=[]  NParamMax=[]  KbParamMin=[]  KbParamMax=[]  KtParamMin=[]  KtParamMax=[]  KbOutMin=[]  KbOutMax=[]  KtOutMin=[]  KtOutMax=[]  IntegratorOutMin=[]  IntegratorOutMax=[]  FilterOutMin=[]  FilterOutMax=[]  SumI1OutMin=[]  SumI1OutMax=[]  SumI2OutMin=[]  SumI2OutMax=[]  SumI3OutMin=[]  SumI3OutMax=[]  SumI4OutMin=[]  SumI4OutMax=[]  SumDOutMin=[]  SumDOutMax=[]  DifferentiatorOutMin=[]  DifferentiatorOutMax=[]  FilterDiffOutCoefMin=[]  FilterDiffOutCoefMax=[]  ReciprocalOutMin=[]  ReciprocalOutMax=[]  SumDenOutMin=[]  SumDenOutMax=[]  SumNumOutMin=[]  SumNumOutMax=[]  DivideOutMin=[]  DivideOutMax=[]  IntegratorContinuousStateAttributes=''  IntegratorStateMustResolveToSignalObject=off  IntegratorRTWStateStorageClass=Auto  FilterContinuousStateAttributes=''  FilterStateMustResolveToSignalObject=off  FilterRTWStateStorageClass=Auto  ParallelPVariant=InternalParameters  IdealPVariant=Disabled  IVariant=InternalParameters  DVariant=InternalParameters  IntegratorVariant=Discrete  SatVariant=Enabled  AWVariant=DiscClampingParallel  PCopyVariant=Disabled  TRVariant=Disabled  FdbkBlocksVariant=Forward  IdealPFdbkVariant=Disabled  SatFdbkVariant=Disabled  DerivativeFilterVariant=ForwardEulerFilter  NVariant=InternalParameters  NCopyVariant=Disabled  FilterICVariant=InternalICsFilter  IntegratorICVariant=InternalICs  ExternalResetVariant=Disabled  TRSumVariant=Passthrough  SumFdbkVariant=Disabled  SumVariant=Sum_PID
  Discrete PID Controller 2 : simulink/Continuous/PID Controller  Controller=PID  Form=Parallel  TimeDomain=Discrete-time  SampleTime=Ctr.TS  IntegratorMethod=Forward Euler  FilterMethod=Forward Euler  ControllerParametersSource=internal  P=0.0957032759552278  I=0.0036993820124705  D=0.00128202697815644  UseFilter=on  N=46.36307138661  TunerSelectOption=Transfer Function Based (PID Tuner App)  InitialConditionSource=internal  InitialConditionForIntegrator=0  InitialConditionForFilter=0  DifferentiatorICPrevScaledInput=0  ExternalReset=none  TrackingMode=off  Kt=1  LimitOutput=on  UpperSaturationLimit=30  LowerSaturationLimit=-30  LinearizeAsGain=off  AntiWindupMode=clamping  Kb=1  POutMin=[]  POutMax=[]  IOutMin=[]  IOutMax=[]  DOutMin=[]  DOutMax=[]  NOutMin=[]  NOutMax=[]  SumOutMin=[]  SumOutMax=[]  SaturationOutMin=[]  SaturationOutMax=[]  PParamMin=[]  PParamMax=[]  IParamMin=[]  IParamMax=[]  DParamMin=[]  DParamMax=[]  NParamMin=[]  NParamMax=[]  KbParamMin=[]  KbParamMax=[]  KtParamMin=[]  KtParamMax=[]  KbOutMin=[]  KbOutMax=[]  KtOutMin=[]  KtOutMax=[]  IntegratorOutMin=[]  IntegratorOutMax=[]  FilterOutMin=[]  FilterOutMax=[]  SumI1OutMin=[]  SumI1OutMax=[]  SumI2OutMin=[]  SumI2OutMax=[]  SumI3OutMin=[]  SumI3OutMax=[]  SumI4OutMin=[]  SumI4OutMax=[]  SumDOutMin=[]  SumDOutMax=[]  DifferentiatorOutMin=[]  DifferentiatorOutMax=[]  FilterDiffOutCoefMin=[]  FilterDiffOutCoefMax=[]  ReciprocalOutMin=[]  ReciprocalOutMax=[]  SumDenOutMin=[]  SumDenOutMax=[]  SumNumOutMin=[]  SumNumOutMax=[]  DivideOutMin=[]  DivideOutMax=[]  IntegratorContinuousStateAttributes=''  IntegratorStateMustResolveToSignalObject=off  IntegratorRTWStateStorageClass=Auto  FilterContinuousStateAttributes=''  FilterStateMustResolveToSignalObject=off  FilterRTWStateStorageClass=Auto  ParallelPVariant=InternalParameters  IdealPVariant=Disabled  IVariant=InternalParameters  DVariant=InternalParameters  IntegratorVariant=Discrete  SatVariant=Enabled  AWVariant=DiscClampingParallel  PCopyVariant=Disabled  TRVariant=Disabled  FdbkBlocksVariant=Forward  IdealPFdbkVariant=Disabled  SatFdbkVariant=Disabled  DerivativeFilterVariant=ForwardEulerFilter  NVariant=InternalParameters  NCopyVariant=Disabled  FilterICVariant=InternalICsFilter  IntegratorICVariant=InternalICs  ExternalResetVariant=Disabled  TRSumVariant=Passthrough  SumFdbkVariant=Disabled  SumVariant=Sum_PID
  Fcn2 : Fcn  Expr=0.5 * u(1)^2
  Fcn4 : Fcn  Expr=0.5 * u(1)^2
  Gain1 : Gain  Gain=C.g
  Gain3 : Gain  Gain=C.g
  Selector1 : Selector  InputPortWidth=3  IndexOptions=Index vector (dialog)  Indices=3  OutputSizes=1
  Sum : Sum  Inputs=|++
  Sum11 : Sum  Inputs=+-
  Sum12 : Sum  Inputs=+-
  Sum13 : Sum  Inputs=|-+
  Sum8 : Sum  Inputs=|++
  Sum9 : Sum  Inputs=|-+
  ThrottleDem : Outport  VectorParamsAs1DForOutWhenUnconnected=off
  PitchDem : Outport  Port=2  VectorParamsAs1DForOutWhenUnconnected=off
  wires:
  Discrete PID Controller 2/1 -> PitchDem/1  "pitch"
  Discrete PID Controller 1/1 -> ThrottleDem/1  "throttle"
  [Va] -> Fcn2/1
  Fcn2/1 -> Sum/2, Sum11/2  "SKE"
  PlantData/1 -> Bus Selector1/1
  Bus Selector1/1 -> Selector1/1  "<xyh>"
  Selector1/1 -> Gain1/1
  Gain1/1 -> Sum/1, Sum11/1  "SPE"
  Target_Height/1 -> Gain3/1
  Gain3/1 -> Sum12/1, Sum8/1  "SPE_c"
  Target_Airspeed/1 -> Fcn4/1
  Fcn4/1 -> Sum12/2, Sum8/2  "SKE_c"
  Sum/1 -> Sum9/1  "Specific total energy"
  Sum8/1 -> Sum9/2  "Demanded specific total energy"
  Sum9/1 -> Discrete PID Controller 1/1  "STE err"
  Sum11/1 -> Sum13/1  "Specific energy balance"
  Sum12/1 -> Sum13/2  "Demanded specific energy balance"
  Sum13/1 -> Discrete PID Controller 2/1  "SBE err"

== system Bixler/BIXLER DYNAMICS/Actuator Dynamics ==
  In : Inport
  +-15 : Saturate  UpperLimit=15  LowerLimit=-15
  +-25 : Saturate  UpperLimit=25  LowerLimit=-25
  +-30 : Saturate  UpperLimit=30  LowerLimit=-30
  Bus Creator1 : BusCreator  Inputs='delta_ail','delta_elev','delta_rudd'
  Bus Selector : BusSelector  OutputSignals=ailerons,elevator,rudder
  Scope : Scope  NumInputPorts=2
  Transfer Fcn : TransferFcn  Numerator=[45]  Denominator=[1 45]
  Transfer Fcn1 : TransferFcn  Numerator=[45]  Denominator=[1 45]
  Transfer Fcn2 : TransferFcn  Numerator=[45]  Denominator=[1 45]
  Out : Outport  Unit=deg  VectorParamsAs1DForOutWhenUnconnected=off
  wires:
  +-30/1 -> Bus Creator1/1  "delta_ail"
  Bus Creator1/1 -> Out/1  "ControlActions"
  +-25/1 -> Bus Creator1/3  "delta_rudd"
  +-15/1 -> Bus Creator1/2  "delta_elev"
  Bus Selector/2 -> Transfer Fcn1/1  "<elevator>"
  Bus Selector/1 -> Scope/1, Transfer Fcn/1  "<ailerons>"
  Bus Selector/3 -> Transfer Fcn2/1  "<rudder>"
  In/1 -> Bus Selector/1
  Transfer Fcn/1 -> Scope/2, +-30/1
  Transfer Fcn1/1 -> +-15/1
  Transfer Fcn2/1 -> +-25/1

== system Bixler/BIXLER DYNAMICS/RUBBISH BIN ==
  Angle Conversion1 : aerolibconvert2/Angle Conversion  Commented=on  IU=deg  OU=rad
  Clock : Clock  Commented=on
  Constant1 : Constant  Commented=on  Value=0
  From1 : From  Commented=on  GotoTag=throttle
  From2 : From  Commented=on  GotoTag=Target_Height  TagVisibility=global
  From3 : From  Commented=on  GotoTag=Target_Airspeed  TagVisibility=global
  From7 : From  Commented=on  GotoTag=throttle
  From9 : From  Commented=on  GotoTag=PlantData
  Orbit : Subsystem  Commented=on
  Reference Signals : Subsystem  Commented=on
  Reference Signals1 : Subsystem  Commented=on
  Straight Line : Subsystem  Commented=on
  Switch : Switch  Commented=on  Criteria=u2 > Threshold  Threshold=50
  TECS : Subsystem  Commented=on
  Vector Field : MATLAB Function  Commented=on  TreatAsAtomicUnit=on
  wires:
  From7/1 -> Reference Signals/1(Throttle)
  Clock/1 -> Switch/2
  Constant1/1 -> Angle Conversion1/1
  Angle Conversion1/1 -> Switch/3
  Vector Field/1(y) -> Switch/1
  From1/1 -> Reference Signals1/1(Throttle)
  From2/1 -> TECS/3(HeightDemand)
  From3/1 -> TECS/2(TAS_dem)
  From9/1 -> TECS/1(PlantData)

== system Bixler/BIXLER DYNAMICS/Sampling ==
  Cont. : Inport
  Bus Creator : BusCreator  Inputs=1
  Cont.+Disc. : Outport  VectorParamsAs1DForOutWhenUnconnected=off
  wires:
  Cont./1 -> Bus Creator/1  "PlantData"
  Bus Creator/1 -> Cont.+Disc./1

== system Bixler/BIXLER DYNAMICS/Sampling  ==
  Cont. : Inport
  Bus Creator : BusCreator  Inputs=1
  Cont.+Disc. : Outport  VectorParamsAs1DForOutWhenUnconnected=off
  wires:
  Bus Creator/1 -> Cont.+Disc./1
  Cont./1 -> Bus Creator/1  "DerCond"

== system Bixler/BIXLER DYNAMICS/Throttle Dynamics ==
  In : Inport  Unit=%
  0-100 : Saturate  UpperLimit=100  LowerLimit=0
  Transfer Fcn2 : TransferFcn  Numerator=[45]  Denominator=[1 45]
  Out : Outport  Unit=%  VectorParamsAs1DForOutWhenUnconnected=off
  wires:
  In/1 -> Transfer Fcn2/1
  0-100/1 -> Out/1
  Transfer Fcn2/1 -> 0-100/1

== system Bixler/BIXLER DYNAMICS/Vehicle Airframe ==
  Throttle_cmd : Inport  Unit=%
  ControlActions : Inport  Port=2
  EnvData : Inport  Port=3
  6DOF (Euler Angles) : shared6dof/6DOF (Euler Angles)  units=Metric (MKS)  mtype=Fixed  rep=Euler Angles  xme_0=Init.xyz  Vm_0=Init.uvw  eul_0=deg2rad(Init.attitude)  pm_0=deg2rad(Init.pqr)  mass_0=Bxl.mass  mass_e=0.5  mass_f=2.0  inertia=Bxl.J  inertia_e=eye(3)  inertia_f=2*eye(3)  k_quat=1.0  vre_flag=on  abi_flag=off  aMode=aMode  xme_statename=''  Vm_statename=''  eul_statename=''  quat_statename=''  pm_statename=''  mass_statename=''
      settings: SourceProductBaseCode=AE,PW,DR,MT,UV,VE
  Aerodynamics : Subsystem
  Bus Creator : BusCreator  Inputs=13
  Bus Creator1 : BusCreator  Inputs='qbar','alpha','beta','Va','Course','CrabAngle','WAE'
  Bus Creator2 : BusCreator  Inputs=2
  Bus Creator3 : BusCreator  Inputs=4
  Derived Conditions : Subsystem
  Ed : MATLAB Function  TreatAsAtomicUnit=on
  Ed1 : MATLAB Function  TreatAsAtomicUnit=on
  Ed2 : MATLAB Function  TreatAsAtomicUnit=on
  Gain : Gain  Gain=[1 1 -1]
  Gravity Force : Subsystem
  Propulsion : Subsystem
  Scope : Scope
  Scope1 : Scope
  Scope2 : Scope
  Sum : Sum
  Sum1 : Sum  Inputs=+++|
  inv : MATLAB Function  TreatAsAtomicUnit=on
  to Omega_e : Subsystem
  PlantData : Outport  VectorParamsAs1DForOutWhenUnconnected=off
  DerCond : Outport  Port=2  VectorParamsAs1DForOutWhenUnconnected=off
  tag scope: in2=global, in=global
  wires:
  [DCM] -> inv/1(u), Bus Creator/7  "From inertial to body matrix"
  [euler] -> Ed2/3(attitude), Ed/1(attitude), to Omega_e/1(euler), Bus Creator/4  "Euler angles (rad)"
  [Vb] -> Ed1/1(Vb), Bus Creator/8  "Velocity (body)"
  [PlantData] -> Derived Conditions/2(PlantData)
  EnvData/1 -> Derived Conditions/1(EnvData)
  [PlantData] -> Aerodynamics/1(PlantData)
  [Ve] -> Bus Creator/1  "Velocity (inertial)"
  [Xe] -> Gain/1, Bus Creator/2  "Position (inertial)"
  [A_b] -> Bus Creator/10, Ed1/2(Ab)  "Accelerations (body/body)"
  ControlActions/1 -> Bus Creator2/2, Aerodynamics/3(Control)
  Sum1/1 -> 6DOF (Euler Angles)/1
  Bus Creator/1 -> PlantData/1, [PlantData]
  Sum/1 -> 6DOF (Euler Angles)/2
  Bus Creator1/1 -> [DerCond], DerCond/1
  [PlantData] -> Gravity Force/1(PlantData)
  Gravity Force/1(Fg) -> Sum1/1
  Derived Conditions/1(qbar) -> Bus Creator1/1  "qbar"
  Derived Conditions/2(alpha) -> Bus Creator1/2  "alpha"
  Derived Conditions/4(Va) -> Bus Creator1/4  "Va"
  Derived Conditions/3(beta) -> Bus Creator1/3  "beta"
  Throttle_cmd/1 -> Bus Creator2/1, Propulsion/1(Throttle)
  Propulsion/2(M) -> Sum/1, Bus Creator3/2
  Propulsion/1(F) -> Sum1/2, Bus Creator3/1
  [DerCond] -> Aerodynamics/2(DerCond)
  Aerodynamics/1(AeroForces) -> Bus Creator3/3, Sum1/3
  Aerodynamics/2(AeroMoments) -> Bus Creator3/4, Sum/2
  [ome_d_b] -> Ed2/2(omeb_d), Bus Creator/9  "Angular accelerations (body/body)"
  [ome_b] -> Bus Creator/6, Ed/2(ome_b), Ed2/1(omeb), to Omega_e/2(ome_b)  "Angular rates (body) (rad/s)"
  Gain/1 -> Bus Creator/3  "xyh"
  Derived Conditions/5(CourseAngle) -> Bus Creator1/5  "Course"
  Derived Conditions/6(CrabAngle) -> Bus Creator1/6  "CrabAngle"
  Derived Conditions/7(WAE) -> Bus Creator1/7  "WAE"
  to Omega_e/1(ome_e) -> Ed1/4(ome_e), Ed2/4(omee), Scope2/1, Bus Creator/5  "ome_e"
  6DOF (Euler Angles)/1 -> [Ve]
  6DOF (Euler Angles)/2 -> Scope/1, [Xe]
  6DOF (Euler Angles)/3 -> Scope1/1, [euler]
  6DOF (Euler Angles)/4 -> [DCM]
  6DOF (Euler Angles)/5 -> [Vb]
  6DOF (Euler Angles)/6 -> [ome_b]
  6DOF (Euler Angles)/7 -> [ome_d_b]
  6DOF (Euler Angles)/8 -> [A_b]
  [DerCond] -> Propulsion/2(DerCond)
  Ed/1(ome_e) -> Bus Creator/11  "Ed"
  Bus Creator2/1 -> [in]
  Bus Creator3/1 -> [in2]
  Ed1/1(Ae) -> Bus Creator/12  "Ae"
  inv/1(y) -> Ed1/3(Rb_e)
  Ed2/1(Edd) -> Bus Creator/13  "Edd"
